simulink model "problem_c"  (R2022a)
settings: Solver=VariableStepAuto  StartTime=0.0  StopTime=0.14  RelTol=1e-3
settings Model: Creator=13269  LastModifiedBy=13269

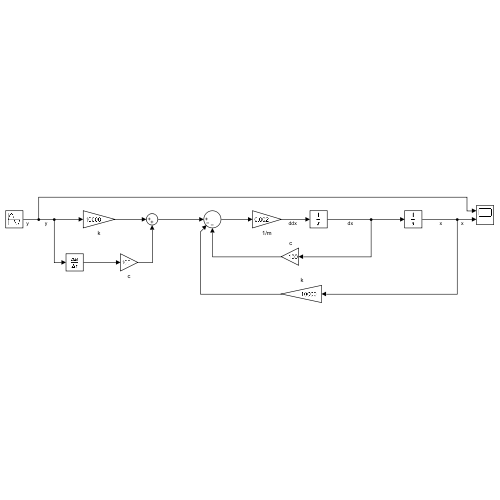
[thumbnail: Simulink's stored preview of the top-level diagram]
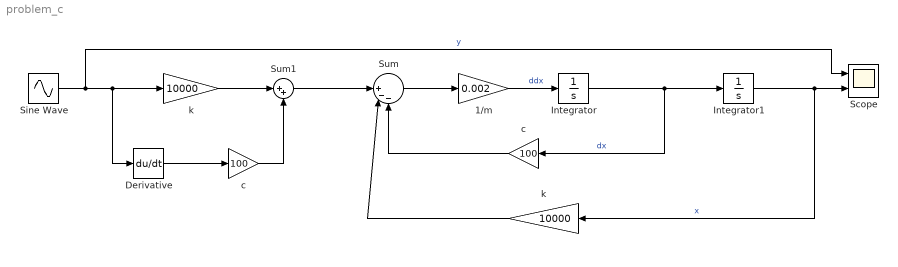
== system problem_c ==
  " c" : Gain  Gain=100
  " k" : Gain  Gain=10000
  1/m : Gain  Gain=0.002
  Derivative : Derivative
  Integrator : Integrator
  Integrator1 : Integrator
  Scope : Scope  NumInputPorts=2
  Sine Wave : Sin  Amplitude=-0.375  Bias=-0.08  Frequency=22.22  SampleTime=0
  Sum : Sum  Inputs=||+--
  Sum1 : Sum  Inputs=|++
  c : Gain  Gain=100
  k : Gain  Gain=10000
  wires:
  1/m/1 -> Integrator/1  "ddx"
  Integrator/1 -> " c"/1, Integrator1/1  "dx"
  Integrator1/1 -> " k"/1, Scope/2  "x"
  k/1 -> Sum1/1
  Sine Wave/1 -> Derivative/1, k/1, Scope/1  "y"
  Sum1/1 -> Sum/1
  c/1 -> Sum1/2
  Sum/1 -> 1/m/1
  " c"/1 -> Sum/3
  " k"/1 -> Sum/2
  Derivative/1 -> c/1
